simulink model "solve_algebraic_equations"  (R2021a)
settings: Solver=VariableStepAuto  StartTime=0.0  StopTime=10.0  RelTol=1e-3
settings Model: Creator=DELL  LastModifiedBy=DELL

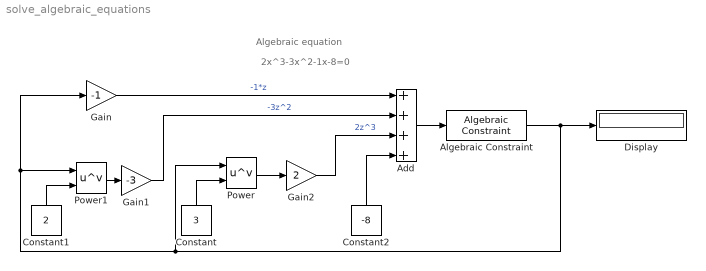
== system solve_algebraic_equations ==
  note: 2x^3-3x^2-1x-8=0
  note: Algebraic equation
  Add : Sum  Inputs=++++
  Algebraic Constraint : AlgebraicConstraint
  Constant : Constant  Value=3
  Constant1 : Constant  Value=2
  Constant2 : Constant  Value=-8
  Display : Display
  Gain : Gain  Gain=-1
  Gain1 : Gain  Gain=-3
  Gain2 : Gain  Gain=2
  Power : Math  Operator=pow  SaturateOnIntegerOverflow=on
  Power1 : Math  Operator=pow  SaturateOnIntegerOverflow=on
  wires:
  Algebraic Constraint/1 -> Display/1, Gain/1, Power1/1, Power/1
  Constant/1 -> Power/2
  Constant1/1 -> Power1/2
  Add/1 -> Algebraic Constraint/1
  Gain/1 -> Add/1  "-1*z"
  Power1/1 -> Gain1/1
  Gain1/1 -> Add/2  "-3z^2"
  Power/1 -> Gain2/1
  Gain2/1 -> Add/3  "2z^3"
  Constant2/1 -> Add/4
